simulink model "systemsim"  (R2016a)
settings: Solver=VariableStepAuto  StartTime=0.0  StopTime=simtime  RelTol=1e-3
values from neighbouring files (symbols this model uses):
  Ki = 1/Ti    (= 0.000694444444444)    [simulation.m]
  Kp = -150    [simulation.m]
  steptime = 600    [simulation.m]
  sys = n4sid(data,nx)    [identification.m]    (also in identification_general.m = n4sid(data,nx, 'inputdelay', 60); simulation.m = n4sid(data,nx, 'inputdelay',delay))
  Ts = 1    [identification.m]    (also in identification_general.m; simulation.m)
libraries: simulink x1
settings Model: Creator=Sondre  LastModifiedBy=Sondre

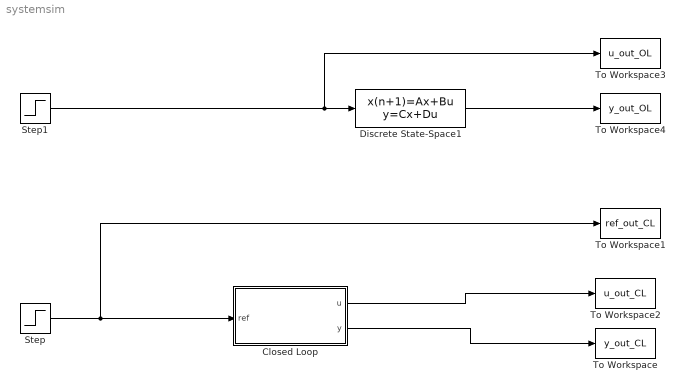
== system systemsim ==
  "Closed Loop " : Subsystem
  Discrete State-Space1 : DiscreteStateSpace  A=sys.A  B=sys.B  C=sys.C  D=sys.D  SampleTime=Ts
  Step : Step  Time=steptime  SampleTime=0
  Step1 : Step  Time=steptime  SampleTime=0
  To Workspace : ToWorkspace  VariableName=y_out_CL  SaveFormat=Timeseries  SampleTime=-1
  To Workspace1 : ToWorkspace  VariableName=ref_out_CL  SaveFormat=Timeseries  SampleTime=-1
  To Workspace2 : ToWorkspace  VariableName=u_out_CL  SaveFormat=Timeseries  SampleTime=-1
  To Workspace3 : ToWorkspace  VariableName=u_out_OL  SaveFormat=Timeseries  SampleTime=-1
  To Workspace4 : ToWorkspace  VariableName=y_out_OL  SaveFormat=Timeseries  SampleTime=-1
  wires:
  Step/1 -> "Closed Loop "/1(ref), To Workspace1/1
  "Closed Loop "/1("u ") -> To Workspace2/1
  "Closed Loop "/2(y) -> To Workspace/1
  Step1/1 -> Discrete State-Space1/1, To Workspace3/1
  Discrete State-Space1/1 -> To Workspace4/1

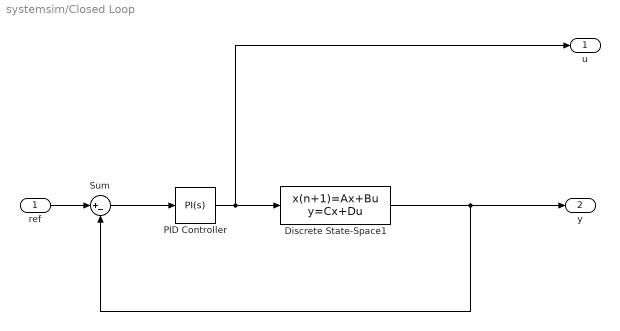
== system systemsim/Closed Loop  ==
  ref : Inport
  Discrete State-Space1 : DiscreteStateSpace  A=sys.A  B=sys.B  C=sys.C  D=sys.D  SampleTime=Ts
  PID Controller : simulink/Continuous/PID Controller  Controller=PI  TimeDomain=Continuous-time  SampleTime=-1  IntegratorMethod=Forward Euler  FilterMethod=Forward Euler  Form=Ideal  UseFilter=on  ControllerParametersSource=internal  P=Kp  I=Ki  D=0  N=100  InitialConditionSource=internal  InitialConditionForIntegrator=0  InitialConditionForFilter=0  ExternalReset=none  LimitOutput=off  UpperSaturationLimit=inf  LowerSaturationLimit=-inf  LinearizeAsGain=on  AntiWindupMode=none  Kb=1  TrackingMode=off  Kt=1  PParamMin=[]  PParamMax=[]  IParamMin=[]  IParamMax=[]  DParamMin=[]  DParamMax=[]  NParamMin=[]  NParamMax=[]  KbParamMin=[]  KbParamMax=[]  KtParamMin=[]  KtParamMax=[]  POutMin=[]  POutMax=[]  IOutMin=[]  IOutMax=[]  DOutMin=[]  DOutMax=[]  NOutMin=[]  NOutMax=[]  KbOutMin=[]  KbOutMax=[]  KtOutMin=[]  KtOutMax=[]  IntegratorOutMin=[]  IntegratorOutMax=[]  FilterOutMin=[]  FilterOutMax=[]  SumOutMin=[]  SumOutMax=[]  SumI1OutMin=[]  SumI1OutMax=[]  SumI2OutMin=[]  SumI2OutMax=[]  SumI3OutMin=[]  SumI3OutMax=[]  SumDOutMin=[]  SumDOutMax=[]  SaturationOutMin=[]  SaturationOutMax=[]  IntegratorContinuousStateAttributes=''  IntegratorStateMustResolveToSignalObject=off  IntegratorRTWStateStorageClass=Auto  FilterContinuousStateAttributes=''  FilterStateMustResolveToSignalObject=off  FilterRTWStateStorageClass=Auto  DifferentiatorICPrevScaledInput=0  DifferentiatorOutMin=[]  DifferentiatorOutMax=[]
  Sum : Sum  Inputs=|+-
  "u " : Outport
  y : Outport  Port=2
  wires:
  Sum/1 -> PID Controller/1
  PID Controller/1 -> "u "/1, Discrete State-Space1/1
  Discrete State-Space1/1 -> y/1, Sum/2
  ref/1 -> Sum/1
